simulink model "quadcopter_nonlinear_continuous"  (R2019a)
settings: Solver=VariableStepAuto  StartTime=0.0  StopTime=20  RelTol=1e-3
undefined symbols (not defined in the file): sigbuilder_block
settings Model: Creator=vardhah  LastModifiedBy=vardhah

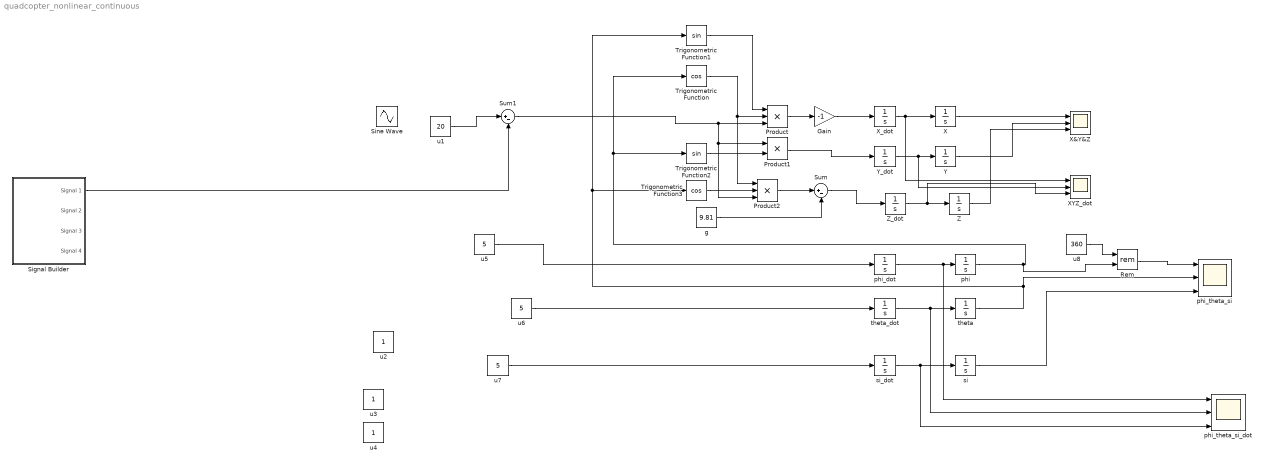
== system quadcopter_nonlinear_continuous ==
  Gain : Gain  Gain=-1
  Product : Product  Inputs=3
  Product1 : Product
  Product2 : Product  Inputs=3
  Rem : Math  Operator=rem  SaturateOnIntegerOverflow=on
  Signal Builder : Subsystem  Tag=STV Subsys  LoadFcn=sigbuilder_block('load');  StartFcn=sigbuilder_block('start');  StopFcn=sigbuilder_block('stop');  ClipboardFcn=sigbuilder_block('clipboard');  mask(Sigbuilder block){tuvar=[0:10]}
      mask help: Simulink:masks:SigbuilderBlock_MD
      mask init:
      | if ~strcmp(get_param(bdroot(gcbh),'SimulationStatus'),'stopped') tuvar = sigbuilder_block('maskInit'); end
      settings: CopyFcn=sigbuilder_block('copy');  DeleteFcn=sigbuilder_block('delete');  ModelCloseFcn=sigbuilder_block('modelClose');  PreSaveFcn=sigbuilder_block('preSave');  PauseFcn=sigbuilder_block('pause');  ContinueFcn=sigbuilder_block('continue');  NameChangeFcn=sigbuilder_block('namechange');  OpenFcn=sigbuilder_block('open',[43.5 30.75 550.5 399.75 ]);  CloseFcn=sigbuilder_block('close');
      mask Display: plot(0, 0, 100, 100,[2, 2, 32, 32, 2], [68, 8, 8, 68, 68],[32, 2], [38, 38], [32, 19, 2],[53, 60, 44], [32, 17, 17, 2],[16, 16, 31, 31]);txt = getActiveGroup(gcbh);text(2, 100, txt,'verticalAlignment', 'top');
  Sine Wave : Sin  SampleTime=0
  Sum : Sum  Inputs=|+-
  Sum1 : Sum  Inputs=|+-
  Trigonometric Function : Trigonometry  Operator=cos
  Trigonometric Function1 : Trigonometry
  Trigonometric Function2 : Trigonometry
  Trigonometric Function3 : Trigonometry  Operator=cos
  X : Integrator
  X&Y&Z : Scope  NumInputPorts=3
  "XYZ_dot " : Scope  NumInputPorts=3
  X_dot : Integrator
  Y : Integrator
  Y_dot : Integrator
  Z : Integrator
  Z_dot : Integrator
  g : Constant  Value=9.81
  phi : Integrator
  phi_dot : Integrator
  "phi_theta_si " : Scope  NumInputPorts=3
  phi_theta_si_dot : Scope  NumInputPorts=3
  si : Integrator
  si_dot : Integrator
  theta : Integrator
  theta_dot : Integrator
  u1 : Constant  Value=20
  u2 : Constant
  u3 : Constant
  u4 : Constant
  u5 : Constant  Value=5
  u6 : Constant  Value=5
  u7 : Constant  Value=5
  u8 : Constant  Value=360
  wires:
  Trigonometric Function/1 -> Product2/1, Product/2
  Trigonometric Function1/1 -> Product/1
  Product/1 -> Gain/1
  Trigonometric Function2/1 -> Product1/2
  Gain/1 -> X_dot/1
  X_dot/1 -> "XYZ_dot "/1, X/1
  Y_dot/1 -> "XYZ_dot "/2, Y/1
  Product1/1 -> Y_dot/1
  Trigonometric Function3/1 -> Product2/2
  Product2/1 -> Sum/1
  g/1 -> Sum/2
  Sum/1 -> Z_dot/1
  Z_dot/1 -> "XYZ_dot "/3, Z/1
  phi_dot/1 -> phi_theta_si_dot/1, phi/1
  phi/1 -> Rem/2, Trigonometric Function2/1, Trigonometric Function/1
  theta/1 -> Trigonometric Function3/1, Trigonometric Function1/1, "phi_theta_si "/2
  theta_dot/1 -> phi_theta_si_dot/2, theta/1
  si/1 -> "phi_theta_si "/3
  si_dot/1 -> phi_theta_si_dot/3, si/1
  X/1 -> X&Y&Z/1
  Y/1 -> X&Y&Z/2
  Z/1 -> X&Y&Z/3
  Signal Builder/1(Signal 1) -> Sum1/2
  Sum1/1 -> Product2/3, Product1/1, Product/3
  u5/1 -> phi_dot/1
  u6/1 -> theta_dot/1
  u7/1 -> si_dot/1
  u1/1 -> Sum1/1
  u8/1 -> Rem/1
  Rem/1 -> "phi_theta_si "/1

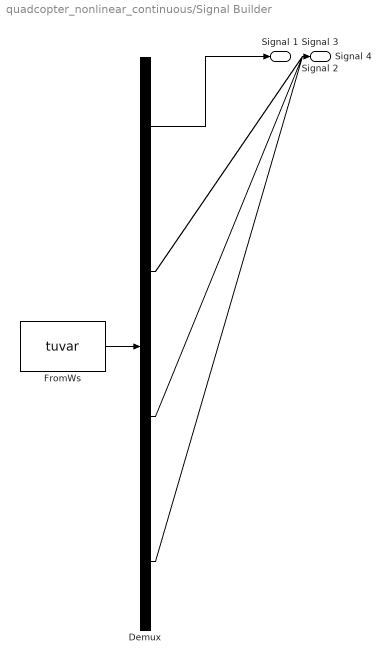
== system quadcopter_nonlinear_continuous/Signal Builder ==
  Demux : Demux  Tag=STV Demux
  FromWs : FromWorkspace  Tag=STV FromWs  VariableName=tuvar  SampleTime=0
      SigBuilderData=|
      | common.afterFinalStr = 'Extrapolate'
      | common.sampleTime = 0
      | dataSet.timeRange = [0 10]
      | dataSet.name = 'Group 1'
      | sbobj.Groups.Name = 'Group 1'
      | sbobj.Groups.Signals(1).Name = 'Signal 1'
      | sbobj.Groups.Signals(1).XData = [0 4 4 6 6 10]
      | sbobj.Groups.Signals(1).YData = [0 0 1 1 0 0]
      | sbobj.Groups.Signals(2).Name = 'Signal 2'
      | sbobj.Groups.Signals(2).XData = [0 4 4 6 6 10]
      | sbobj.Groups.Signals(2).YData = [0 0 1 1 0 0]
      | sbobj.Groups.Signals(3).Name = 'Signal 3'
      | sbobj.Groups.Signals(3).XData = [0 4 4 6 6 10]
      | sbobj.Groups.Signals(3).YData = [0 0 1 1 0 0]
      | sbobj.Groups.Signals(4).Name = 'Signal 4'
      | sbobj.Groups.Signals(4).XData = [0 4 4 6 6 10]
      | sbobj.Groups.Signals(4).YData = [0 0 1 1 0 0]
  Signal 1 : Outport  Tag=STV Outport
  Signal 2 : Outport  Tag=STV Outport  Port=2
  Signal 3 : Outport  Tag=STV Outport  Port=3
  Signal 4 : Outport  Tag=STV Outport  Port=4
  wires:
  Demux/1 -> Signal 1/1
  FromWs/1 -> Demux/1
  Demux/2 -> Signal 2/1
  Demux/3 -> Signal 3/1
  Demux/4 -> Signal 4/1
